simulink model "vacc_reorder"  (R2021a)
settings: Solver=VariableStepAuto  StartTime=0.0  StopTime=32*4*4+50  RelTol=1e-3
libraries: xbsIndex_r4 x285, casper_library_misc x2, casper_library_delays x2
(part 1 of 2)
settings Model: Creator=jackh  LastModifiedBy=vivado

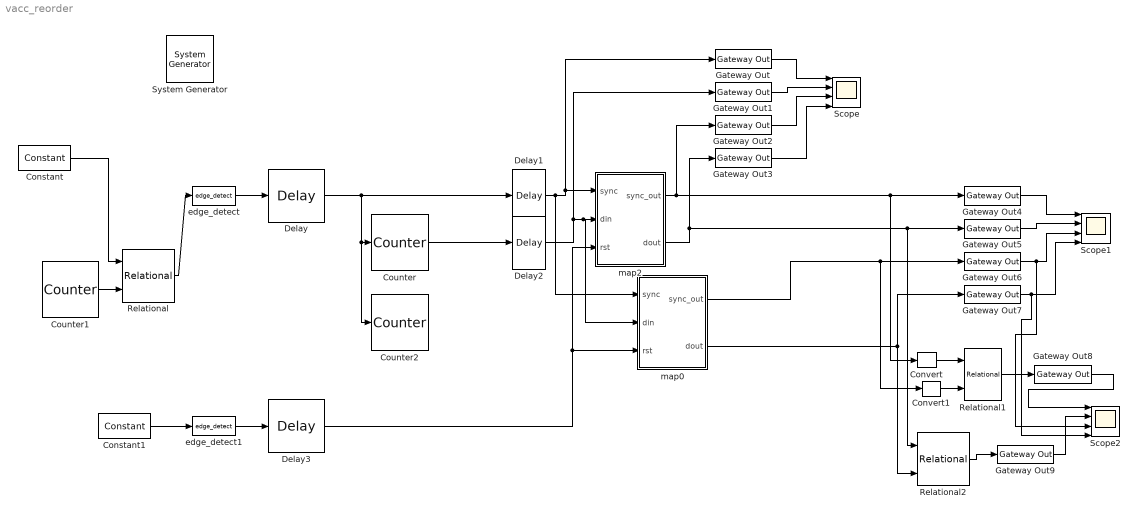
== system vacc_reorder ==
  " System Generator" : xbsIndex_r4/ System Generator  Tag=genX  xilinxfamily=zynquplusRFSOC  part=xczu47dr  speed=-2-e  package=ffvg1517  synthesis_tool=XST  clock_wrapper=Clock Enables  directory=/home/jackh/src/souk-firmware2/souk-firmware/firmware/src/souk_single_pipeline_krm/sysgen  proj_type=Vivado  Synth_file=Vivado Synthesis Defaults  Impl_file=Vivado Implementation Defaults  testbench=off  simulink_period=1  sysclk_period=3.2552  dcm_input_clock_period=10  incr_netlist=off  trim_vbits=Everywhere in SubSystem  dbl_ovrd=According to Block Masks  core_generation=According to Block Masks  run_coregen=off  deprecated_control=off  eval_field=0  block_type=sysgen
  Constant : xbsIndex_r4/Constant  const=0  gui_display_data_type=Fixed-point  arith_type=Unsigned  n_bits=7  bin_pt=0  preci_type=Single  exp_width=8  frac_width=24  explicit_period=on  period=1  equ=P=C  opselect=C  inp2=PCIN>>17  opr=+  inp1=P  carry=CIN  dbl_ovrd=off  block_type=constant
  Constant1 : xbsIndex_r4/Constant  const=1.0  gui_display_data_type=Boolean  arith_type=Boolean  n_bits=16  bin_pt=14  preci_type=Single  exp_width=8  frac_width=24  explicit_period=on  period=1  equ=P=C  opselect=C  inp2=PCIN>>17  opr=+  inp1=P  carry=CIN  dbl_ovrd=off  block_type=constant
  Convert : xbsIndex_r4/Convert  gui_display_data_type=Fixed-point  arith_type=Unsigned  n_bits=1  bin_pt=0  float_type=Single  exp_bits=8  fraction_bits=24  quantization=Truncate  overflow=Wrap  en=off  latency=0  pipeline=off  dbl_ovrd=off  block_type=convert
  Convert1 : xbsIndex_r4/Convert  gui_display_data_type=Fixed-point  arith_type=Unsigned  n_bits=1  bin_pt=0  float_type=Single  exp_bits=8  fraction_bits=24  quantization=Truncate  overflow=Wrap  en=off  latency=0  pipeline=off  dbl_ovrd=off  block_type=convert
  Counter : xbsIndex_r4/Counter  cnt_type=Count Limited  cnt_to=2^5 - 1  operation=Up  start_count=0  cnt_by_val=1  arith_type=Unsigned  n_bits=18*2*4  bin_pt=0  load_pin=off  rst=on  en=off  explicit_period=on  period=1  use_behavioral_HDL=off  implementation=Fabric  dbl_ovrd=off  block_type=counter
  Counter1 : xbsIndex_r4/Counter  cnt_type=Free Running  cnt_to=2^5 - 1  operation=Up  start_count=0  cnt_by_val=1  arith_type=Unsigned  n_bits=7  bin_pt=0  load_pin=off  rst=off  en=off  explicit_period=on  period=1  use_behavioral_HDL=off  implementation=Fabric  dbl_ovrd=off  block_type=counter
  Counter2 : xbsIndex_r4/Counter  cnt_type=Count Limited  cnt_to=0  operation=Down  start_count=2^6 - 1  cnt_by_val=1  arith_type=Unsigned  n_bits=18*2*4  bin_pt=0  load_pin=off  rst=on  en=off  explicit_period=on  period=1  use_behavioral_HDL=off  implementation=Fabric  dbl_ovrd=off  block_type=counter
  Delay : xbsIndex_r4/Delay  rst=off  infoeditControl=Selection of Reset will increase slice count due to use of real FFs and instead of SRLs  en=off  latency=50  reg_retiming=off  dbl_ovrd=off  block_type=delay
  Delay1 : xbsIndex_r4/Delay  rst=off  infoeditControl=Selection of Reset will increase slice count due to use of real FFs and instead of SRLs  en=off  latency=1  reg_retiming=off  dbl_ovrd=off  block_type=delay
  Delay2 : xbsIndex_r4/Delay  rst=off  infoeditControl=Selection of Reset will increase slice count due to use of real FFs and instead of SRLs  en=off  latency=1  reg_retiming=off  dbl_ovrd=off  block_type=delay
  Delay3 : xbsIndex_r4/Delay  rst=off  infoeditControl=Selection of Reset will increase slice count due to use of real FFs and instead of SRLs  en=off  latency=1  reg_retiming=off  dbl_ovrd=off  block_type=delay
  Gateway Out{,1..9} (10 alike) : xbsIndex_r4/Gateway Out  inherit_from_input=off  hdl_port=off  rows=1  columns=1  UseAsDAC=off  DACChannel='1'  interface=None  automatic_assignment=on  address_offset=hex2dec('00')  intf_name=''  intf_description=''  timing_constraint=None  locs_specified=off  LOCs={}  io_standard={}  block_type=gatewayout
  Relational : xbsIndex_r4/Relational  mode=a=b  op_type=Bool  en=off  latency=1  dbl_ovrd=off  block_type=relational
  Relational1 : xbsIndex_r4/Relational  mode=a=b  op_type=Bool  en=off  latency=0  dbl_ovrd=off  block_type=relational
  Relational2 : xbsIndex_r4/Relational  mode=a=b  op_type=Bool  en=off  latency=0  dbl_ovrd=off  block_type=relational
  Scope : Scope  NumInputPorts=4
  Scope1 : Scope  NumInputPorts=4
  Scope2 : Scope  NumInputPorts=4
  edge_detect : casper_library_misc/edge_detect  edge=Rising  polarity=Active High  x_in=[0 0.08 0.08 0.16 0.16 0.24 0.24 0.32 0.32 0.4]  y_in="[-1 -1  1  1  1  1  1  1  1  1]"  x_out=[0.6 0.68 0.68 0.76 0.76 0.84 0.84 0.92 0.92 1]  y_out="[-1 -1  1  1 -1 -1 -1 -1 -1 -1]"
  edge_detect1 : casper_library_misc/edge_detect  edge=Rising  polarity=Active High  x_in=[0 0.08 0.08 0.16 0.16 0.24 0.24 0.32 0.32 0.4]  y_in="[-1 -1  1  1  1  1  1  1  1  1]"  x_out=[0.6 0.68 0.68 0.76 0.76 0.84 0.84 0.92 0.92 1]  y_out="[-1 -1  1  1 -1 -1 -1 -1 -1 -1]"
  map0 : Subsystem  mask{vec_len_bits=5, ram_latency=2, sample_width=18, n_samples=4, add_latency=2}
      mask prompts: vec_len_bits "Vector length (2^?)"; ram_latency "Ram Latency"; sample_width "data width per sample"; n_samples "Number of samples per word"; add_latency "Adder latency"
  map2 : Subsystem  mask{vec_len_bits=5, ram_latency=2, sample_width=18, n_samples=4, add_latency=2}
      mask prompts: vec_len_bits "Vector length (2^?)"; ram_latency "Ram Latency"; sample_width "data width per sample"; n_samples "Number of samples per word"; add_latency "Adder latency"
  wires:
  edge_detect/1 -> Delay/1
  Delay/1 -> Counter2/1, Counter/1, Delay1/1
  Gateway Out1/1 -> Scope/2
  Gateway Out/1 -> Scope/1
  Gateway Out2/1 -> Scope/3
  Gateway Out3/1 -> Scope/4
  Counter1/1 -> Relational/2
  Relational/1 -> edge_detect/1
  Constant/1 -> Relational/1
  Delay1/1 -> map0/1(sync), map2/1(sync), Gateway Out/1
  Delay2/1 -> map0/2(din), map2/2(din), Gateway Out1/1
  Counter/1 -> Delay2/1
  Delay3/1 -> map0/3(rst), map2/3(rst)
  edge_detect1/1 -> Delay3/1
  Constant1/1 -> edge_detect1/1
  Gateway Out7/1 -> Scope2/4, Scope1/4
  Gateway Out6/1 -> Scope2/3, Scope1/3
  Gateway Out4/1 -> Scope1/1
  Gateway Out5/1 -> Scope1/2
  map2/1(sync_out) -> Gateway Out4/1, Convert/1, Gateway Out2/1
  map2/2(dout) -> Relational2/1, Gateway Out5/1, Gateway Out3/1
  Relational1/1 -> Gateway Out8/1
  Gateway Out8/1 -> Scope2/1
  Relational2/1 -> Gateway Out9/1
  Gateway Out9/1 -> Scope2/2
  Convert/1 -> Relational1/1
  Convert1/1 -> Relational1/2
  map0/2(dout) -> Gateway Out7/1, Relational2/2
  map0/1(sync_out) -> Convert1/1, Gateway Out6/1

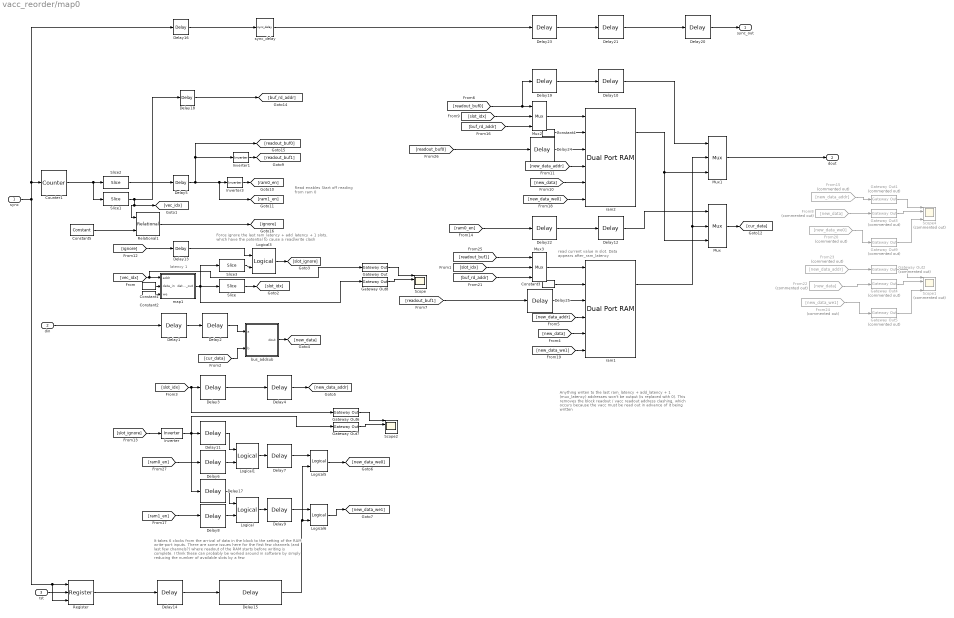
== system vacc_reorder/map0 ==
  note: Force ignore the last ram_latency + add_latency + 1 slots,
      | which have the potential to cause a read/write clash
  note: Anything writen to the last
      | ram_latency + add_latency + 1 (mux_latency)
      | addresses won't be output (is replaced with 0).
      | This removes the block readout / vacc readout address clashing,
      | which occurs because the vacc must be read out in advance of
      | it being written
  note: It takes 6 clocks from the arrival of data in the block
      | to the setting of the RAM write-port inputs. There are some issues
      | here for the first few channels (and last few channels?) where readout
      | of the RAM starts before writing is complete. I think these can probably
      | be worked around in software by simply reducing the number of available
      | slots by a few
  note: Read enables
      | Start off reading from ram 0
  note: read current value in slot.
      | Data appears after_ram_latency
  note: latency 1
  sync : Inport
  din : Inport  Port=2
  rst : Inport  Port=3
  Constant1 : xbsIndex_r4/Constant  const=0  gui_display_data_type=Fixed-point  arith_type=Unsigned  n_bits=32  bin_pt=0  preci_type=Single  exp_width=8  frac_width=24  explicit_period=on  period=1  equ=P=C  opselect=C  inp2=PCIN>>17  opr=+  inp1=P  carry=CIN  dbl_ovrd=off  block_type=constant
  Constant2 : xbsIndex_r4/Constant  const=0  gui_display_data_type=Boolean  arith_type=Boolean  n_bits=32  bin_pt=0  preci_type=Single  exp_width=8  frac_width=24  explicit_period=on  period=1  equ=P=C  opselect=C  inp2=PCIN>>17  opr=+  inp1=P  carry=CIN  dbl_ovrd=off  block_type=constant
  Constant3 : xbsIndex_r4/Constant  const=0  gui_display_data_type=Fixed-point  arith_type=Unsigned  n_bits=2*sample_width * n_samples  bin_pt=0  preci_type=Single  exp_width=8  frac_width=24  explicit_period=on  period=1  equ=P=C  opselect=C  inp2=PCIN>>17  opr=+  inp1=P  carry=CIN  dbl_ovrd=off  block_type=constant
  Constant4 : xbsIndex_r4/Constant  const=0  gui_display_data_type=Fixed-point  arith_type=Unsigned  n_bits=2*sample_width * n_samples  bin_pt=0  preci_type=Single  exp_width=8  frac_width=24  explicit_period=on  period=1  equ=P=C  opselect=C  inp2=PCIN>>17  opr=+  inp1=P  carry=CIN  dbl_ovrd=off  block_type=constant
  Constant5 : xbsIndex_r4/Constant  const="(2^vec_len_bits - 1) - (ram_latency + add_latency +  1 + 1 + 1+1)"  gui_display_data_type=Fixed-point  arith_type=Unsigned  n_bits=vec_len_bits  bin_pt=0  preci_type=Single  exp_width=8  frac_width=24  explicit_period=on  period=1  equ=P=C  opselect=C  inp2=PCIN>>17  opr=+  inp1=P  carry=CIN  dbl_ovrd=off  block_type=constant
  Counter1 : xbsIndex_r4/Counter  cnt_type=Free Running  cnt_to=Inf  operation=Up  start_count=0  cnt_by_val=1  arith_type=Unsigned  n_bits=vec_len_bits + 1  bin_pt=0  load_pin=off  rst=on  en=off  explicit_period=on  period=1  use_behavioral_HDL=off  implementation=Fabric  dbl_ovrd=off  block_type=counter
  Delay{1,5,13..14,16,18..20,22..25} (12 alike) : xbsIndex_r4/Delay  rst=off  infoeditControl=Selection of Reset will increase slice count due to use of real FFs and instead of SRLs  en=off  latency=1  reg_retiming=on  dbl_ovrd=off  block_type=delay
  Delay10 : xbsIndex_r4/Delay  rst=off  infoeditControl=Selection of Reset will increase slice count due to use of real FFs and instead of SRLs  en=off  latency=ram_latency  reg_retiming=on  dbl_ovrd=off  block_type=delay
  Delay11 : xbsIndex_r4/Delay  rst=off  infoeditControl=Selection of Reset will increase slice count due to use of real FFs and instead of SRLs  en=off  latency=1+1  reg_retiming=off  dbl_ovrd=off  block_type=delay
  Delay12 : xbsIndex_r4/Delay  rst=off  infoeditControl=Selection of Reset will increase slice count due to use of real FFs and instead of SRLs  en=off  latency=ram_latency  reg_retiming=on  dbl_ovrd=off  block_type=delay
  Delay15 : xbsIndex_r4/Delay  rst=off  infoeditControl=Selection of Reset will increase slice count due to use of real FFs and instead of SRLs  en=off  latency=ram_latency + add_latency +1+1  reg_retiming=on  dbl_ovrd=off  block_type=delay
  Delay17 : xbsIndex_r4/Delay  rst=off  infoeditControl=Selection of Reset will increase slice count due to use of real FFs and instead of SRLs  en=off  latency=1+1  reg_retiming=off  dbl_ovrd=off  block_type=delay
  Delay2 : xbsIndex_r4/Delay  rst=off  infoeditControl=Selection of Reset will increase slice count due to use of real FFs and instead of SRLs  en=off  latency=ram_latency+1+1  reg_retiming=on  dbl_ovrd=off  block_type=delay
  Delay21 : xbsIndex_r4/Delay  rst=off  infoeditControl=Selection of Reset will increase slice count due to use of real FFs and instead of SRLs  en=off  latency=ram_latency  reg_retiming=on  dbl_ovrd=off  block_type=delay
  Delay3 : xbsIndex_r4/Delay  rst=off  infoeditControl=Selection of Reset will increase slice count due to use of real FFs and instead of SRLs  en=off  latency=ram_latency+1+1  reg_retiming=on  dbl_ovrd=off  block_type=delay
  Delay4 : xbsIndex_r4/Delay  rst=off  infoeditControl=Selection of Reset will increase slice count due to use of real FFs and instead of SRLs  en=off  latency=add_latency  reg_retiming=on  dbl_ovrd=off  block_type=delay
  Delay6 : xbsIndex_r4/Delay  rst=off  infoeditControl=Selection of Reset will increase slice count due to use of real FFs and instead of SRLs  en=off  latency=1+1  reg_retiming=on  dbl_ovrd=off  block_type=delay
  Delay7 : xbsIndex_r4/Delay  rst=off  infoeditControl=Selection of Reset will increase slice count due to use of real FFs and instead of SRLs  en=off  latency=add_latency  reg_retiming=on  dbl_ovrd=off  block_type=delay
  Delay8 : xbsIndex_r4/Delay  rst=off  infoeditControl=Selection of Reset will increase slice count due to use of real FFs and instead of SRLs  en=off  latency=1+1  reg_retiming=on  dbl_ovrd=off  block_type=delay
  Delay9 : xbsIndex_r4/Delay  rst=off  infoeditControl=Selection of Reset will increase slice count due to use of real FFs and instead of SRLs  en=off  latency=add_latency  reg_retiming=on  dbl_ovrd=off  block_type=delay
  From15 : From  Commented=on  GotoTag=new_data_addr
  From20 : From  Commented=on  GotoTag=new_data_we0
  From22 : From  Commented=on  GotoTag=new_data
  From23 : From  Commented=on  GotoTag=new_data_addr
  From24 : From  Commented=on  GotoTag=new_data_we1
  From8 : From  Commented=on  GotoTag=new_data
  Gateway Out{,6..8} (4 alike) : xbsIndex_r4/Gateway Out  inherit_from_input=off  hdl_port=off  rows=1  columns=1  UseAsDAC=off  DACChannel='1'  interface=None  automatic_assignment=on  address_offset=hex2dec('00')  intf_name=''  intf_description=''  timing_constraint=None  locs_specified=off  LOCs={}  io_standard={}  block_type=gatewayout
  Gateway Out{1..5,9} (6 alike) : xbsIndex_r4/Gateway Out  Commented=on  inherit_from_input=off  hdl_port=off  rows=1  columns=1  UseAsDAC=off  DACChannel='1'  interface=None  automatic_assignment=on  address_offset=hex2dec('00')  intf_name=''  intf_description=''  timing_constraint=None  locs_specified=off  LOCs={}  io_standard={}  block_type=gatewayout
  Inverter : xbsIndex_r4/Inverter  en=off  latency=0  dbl_ovrd=off  block_type=inv
  Inverter1 : xbsIndex_r4/Inverter  en=off  latency=0  dbl_ovrd=off  block_type=inv
  Inverter3 : xbsIndex_r4/Inverter  en=off  latency=0  dbl_ovrd=off  block_type=inv
  Logical : xbsIndex_r4/Logical  logical_function=AND  inputs=2  en=off  latency=ram_latency  precision=Full  arith_type=Unsigned  n_bits=16  bin_pt=0  align_bp=on  dbl_ovrd=off  block_type=logical
  Logical1 : xbsIndex_r4/Logical  logical_function=AND  inputs=2  en=off  latency=ram_latency  precision=Full  arith_type=Unsigned  n_bits=16  bin_pt=0  align_bp=on  dbl_ovrd=off  block_type=logical
  Logical3 : xbsIndex_r4/Logical  logical_function=OR  inputs=2  en=off  latency=0  precision=Full  arith_type=Unsigned  n_bits=16  bin_pt=0  align_bp=on  dbl_ovrd=off  block_type=logical
  Logical5 : xbsIndex_r4/Logical  logical_function=AND  inputs=2  en=off  latency=0  precision=Full  arith_type=Unsigned  n_bits=16  bin_pt=0  align_bp=on  dbl_ovrd=off  block_type=logical
  Logical6 : xbsIndex_r4/Logical  logical_function=AND  inputs=2  en=off  latency=0  precision=Full  arith_type=Unsigned  n_bits=16  bin_pt=0  align_bp=on  dbl_ovrd=off  block_type=logical
  Mux{,1..3} (4 alike) : xbsIndex_r4/Mux  inputs=2  en=off  latency=1  precision=Full  arith_type=Unsigned  n_bits=16  bin_pt=14  quantization=Truncate  overflow=Wrap  dbl_ovrd=off  block_type=mux
  Register : xbsIndex_r4/Register  init=0  rst=on  en=on  dbl_ovrd=off  block_type=register
  Relational1 : xbsIndex_r4/Relational  mode=a>b  op_type=Bool  en=off  latency=0  dbl_ovrd=off  block_type=relational
  Scope : Scope  NumInputPorts=4
  Scope1 : Scope  Commented=on  NumInputPorts=4
  Scope2 : Scope  NumInputPorts=4
  Scope4 : Scope  Commented=on  NumInputPorts=4
  Slice : xbsIndex_r4/Slice  nbits=vec_len_bits  boolean_output=off  mode=Lower Bit Location + Width  bit1=0  base1=MSB of Input  bit0=0  base0=LSB of Input  dbl_ovrd=off  block_type=slice
  Slice1 : xbsIndex_r4/Slice  nbits=vec_len_bits  boolean_output=off  mode=Lower Bit Location + Width  bit1=0  base1=MSB of Input  bit0=0  base0=LSB of Input  dbl_ovrd=off  block_type=slice
  Slice2 : xbsIndex_r4/Slice  nbits=1  boolean_output=on  mode=Lower Bit Location + Width  bit1=0  base1=MSB of Input  bit0=vec_len_bits  base0=LSB of Input  dbl_ovrd=off  block_type=slice
  Slice3 : xbsIndex_r4/Slice  nbits=1  boolean_output=on  mode=Upper Bit Location + Width  bit1=0  base1=MSB of Input  bit0=0  base0=LSB of Input  dbl_ovrd=off  block_type=slice
  bus_addsub : Subsystem  AncestorBlock=casper_library_bus/bus_addsub  mask(bus_addsub){opmode=0, n_bits_a=sample_width*ones(n_samples,1), bin_pt_a=zeros(n_samples,1), type_a=1, n_bits_b=sample_width*ones(n_samples,1), bin_pt_b=zeros(n_samples,1), type_b=1, cmplx=on, misc=off, async=off, floating_point=off, float_type=single, exp_width=6, frac_width=19, n_bits_out=sample_width*ones(n_samples,1), bin_pt_out=zeros(n_samples,1), type_out=1, quantization=0, overflow=1, add_implementation=behavioral HDL, csp_latency=add_latency, pipeline_en=off, pipeline_latency=0}
      mask prompts: opmode "mode (Addition=0, Subtraction=1)"; n_bits_a "a input bit widths"; bin_pt_a "a input binary points"; type_a "a input type (Unsigned=0, Signed=1)"; n_bits_b "b input bit widths"; bin_pt_b "b input binary points"; type_b "b input type (Unsigned=0, Signed=1)"; cmplx "complex"; misc "misc support"; async "asynchronous operation"; floating_point "floating point"; exp_width "exponent width"; frac_width "fraction width"; n_bits_out "output bit widths"; bin_pt_out "output binary points"; type_out "output type (Unsigned=0, Signed=1)"; quantization "quantization strategy (Truncate=0, Round  (unbiased: +/- Inf)=1)"; overflow "overflow strategy (Wrap=0, Saturate=1, Flag as error=2)"; add_implementation "adder implementation"; csp_latency "latency"; pipeline_en "pipeline enable"; pipeline_latency "pipeline latency"
      mask help: Add/subtract components of two busses
      mask init:
      | bus_addsub_init(gcb, ...
      |     'opmode', opmode, ...
      |     'n_bits_a', n_bits_a, ...
      |     'bin_pt_a', bin_pt_a, ...
      |     'type_a', type_a, ...
      |     'n_bits_b', n_bits_b, ...
      |     'bin_pt_b', bin_pt_b, ...
      |     'type_b', type_b, ...
      |     'n_bits_out', n_bits_out, ...
      |     'bin_pt_out', bin_pt_out, ...
      |     'floating_point', floating_point, ...
      |     'float_type', float_type, ...
      |     'exp_width', exp_width, ...
      |     'frac_width', frac_width, ...
      |     'type_out', type_out, ...
      |     'overflow', overflow, ...        
      |     'quantization', quantization, ...
      |     'add_implementation', add_implementation, ...
      |     'csp_latency', csp_latency, ...
      |     'pipeline_en', pipeline_en, ...
      |     'pipeline_latency', pipeline_latency,...
      |     'cmplx', cmplx, ...
      |     'misc', misc, ...
      |     'async', async);
      mask Callback floating_point:
      | onoff = get_param(gcb, 'floating_point');
      | if strcmp(onoff,'on')
      |     enable_fixpt = 'off';
      |     set_param_state(gcb, 'float_type', 'on')
      | 
      |     f_type = get_param(gcb, 'float_type');
      |     if strcmp(f_type,'custom')
      |         set_param_state(gcb, 'exp_width', 'on')
      |         set_param_state(gcb, 'frac_width', 'on')
      |     else
      |         set_param_state(gcb, 'exp_width', 'off')
      |         set_param_state(gcb, 'frac_width', 'off')
      |     end
      | 
      | 
      | else
      |     enable_fixpt = 'on';
      |     set_param_state(gcb, 'float_type', 'off')
      |     set_param_state(gcb, 'exp_width', 'off')
      |     set_param_state(gcb, 'frac_width', 'off')
      | end
      | 
      | set_param_state(gcb, 'n_bits_a', enable_fixpt)
      | set_param_state(gcb, 'bin_pt_a', enable_fixpt)
      | set_param_state(gcb, 'type_a', enable_fixpt)
      | set_param_state(gcb, 'n_bits_b', enable_fixpt)
      | set_param_state(gcb, 'bin_pt_b', enable_fixpt)
      | set_param_state(gcb, 'type_b', enable_fixpt)
      | 
      | set_param_state(gcb, 'n_bits_out', enable_fixpt)
      | set_param_state(gcb, 'bin_pt_out', enable_fixpt)
      | set_param_state(gcb, 'type_out', enable_fixpt)
      | set_param_state(gcb, 'quantization', enable_fixpt)
      | set_param_state(gcb, 'overflow', enable_fixpt)
      mask TypeOptions float_type: single | custom
      mask Callback float_type:
      | f_type = get_param(gcb, 'float_type');
      | if strcmp(f_type,'custom')
      |     set_param_state(gcb, 'exp_width', 'on')
      |     set_param_state(gcb, 'frac_width', 'on')
      | else
      |     set_param_state(gcb, 'exp_width', 'off')
      |     set_param_state(gcb, 'frac_width', 'off')
      | end
      mask TypeOptions add_implementation: behavioral HDL | fabric core | DSP48 core
  map1 : Subsystem  Tag=xps:bram  AncestorBlock=xps_library/Memory/shared_bram  mask{arith_type=Unsigned, addr_width=vec_len_bits, data_width=16, reg_prim_output=off, reg_core_output=off, optimization=Minimum_Area, data_bin_pt=0, init_vals=[2^vec_len_bits-1:-1:0], sample_rate=1, desc_str="", type_desc='uint32'}
      mask prompts: arith_type "Output Data Type"; addr_width "Address width"; data_width "Data Width"; reg_prim_output "Register Primitive Output"; reg_core_output "Register Core Output"; data_bin_pt "Data Binary Point"; init_vals "Initial values (simulation only)"; sample_rate "Sample rate"; desc_str "Description"; type_desc "Data Type Description"
      mask init:
      | shared_bram_mask;
      mask TypeOptions arith_type: Unsigned | Signed  (2's comp)
      mask TypeOptions data_width: 8 | 16 | 32 | 64 | 128 | 256 | 512 | 1024
      mask TypeOptions optimization: Minimum_Area | Low_Power
  ram1 : xbsIndex_r4/Dual Port RAM  depth=2^vec_len_bits  initVector=zeros(1,2^vec_len_bits)  distributed_mem=Block RAM  init_a=0  init_b=0  rst_a=off  rst_b=off  en_a=off  en_b=off  latency=ram_latency  write_mode_A=Read Before Write  write_mode_B=Read Before Write  optimize=Area  dbl_ovrd=off  simulation_type=fast_sim  block_type=dpram
  ram2 : xbsIndex_r4/Dual Port RAM  depth=2^vec_len_bits  initVector=zeros(1,2^vec_len_bits)  distributed_mem=Block RAM  init_a=0  init_b=0  rst_a=off  rst_b=off  en_a=off  en_b=off  latency=ram_latency  write_mode_A=Read Before Write  write_mode_B=Read Before Write  optimize=Area  dbl_ovrd=off  simulation_type=fast_sim  block_type=dpram
  sync_delay : casper_library_delays/sync_delay  DelayLen=2^vec_len_bits
      settings: SourceProductName=CASPER DSP Blockset
  sync_out : Outport
  dout : Outport  Port=2
  wires:
  Delay25/1 -> ram1/3
  Delay24/1 -> ram2/3
  Delay23/1 -> Delay21/1
  Delay22/1 -> Delay12/1
  Delay19/1 -> Delay10/1
  Gateway Out8/1 -> Scope/2
  ? -> Scope/4
  Gateway Out/1 -> Scope/1
  ? -> Scope/3
  Delay18/1 -> [buf_rd_addr]
  From20/1 -> Gateway Out9/1
  From8/1 -> Gateway Out3/1
  From15/1 -> Gateway Out1/1
  Gateway Out9/1 -> Scope4/4
  Gateway Out3/1 -> Scope4/2
  ? -> Scope4/3
  Gateway Out1/1 -> Scope4/1
  Delay16/1 -> sync_delay/1
  Inverter1/1 -> [readout_buf1]
  Relational1/1 -> [ignore]
  Constant5/1 -> Relational1/2
  Inverter3/1 -> [ram0_en]
  map1/1(data_out) -> Slice3/1, Slice/1, Gateway Out8/1
  Counter1/1 -> Slice2/1, Slice1/1
  Slice1/1 -> [vec_idx], Relational1/1, Delay18/1
  [vec_idx] -> map1/1(addr), Gateway Out/1
  Constant1/1 -> map1/2(data_in)
  Constant2/1 -> map1/3(we)
  din/1 -> Delay1/1
  Slice/1 -> [slot_idx]
  Delay1/1 -> Delay2/1
  [cur_data] -> bus_addsub/2(b)
  Delay2/1 -> bus_addsub/1(a)
  Delay3/1 -> Delay4/1
  bus_addsub/1(dout) -> [new_data]
  Delay4/1 -> [new_data_addr]
  Slice2/1 -> Delay5/1
  ram2/1 -> Mux/3, Mux1/3
  [readout_buf0] -> Delay24/1
  Mux/1 -> [cur_data]
  Mux2/1 -> ram2/1
  [buf_rd_addr] -> Mux2/3
  [slot_idx] -> Mux2/2
  [slot_idx] -> Mux3/2
  [buf_rd_addr] -> Mux3/3
  Mux3/1 -> ram1/1
  Constant3/1 -> ram1/2
  Constant4/1 -> ram2/2
  ram1/1 -> Mux1/2, Mux/2
  [ram0_en] -> Delay6/1
  [ram1_en] -> Delay8/1
  [new_data] -> ram1/5
  [new_data_addr] -> ram1/4
  [new_data_we1] -> ram1/6
  [ram0_en] -> Delay22/1
  Delay12/1 -> Mux/1
  [readout_buf1] -> Delay25/1
  Mux1/1 -> dout/1
  Delay20/1 -> sync_out/1
  Delay21/1 -> Delay20/1
  sync_delay/1 -> Delay23/1
  sync/1 -> Register/3, Register/1, Counter1/1, Delay16/1
  [new_data_addr] -> ram2/4
  [new_data_we0] -> ram2/6
  [new_data] -> ram2/5
  [slot_ignore] -> Inverter/1
  Inverter/1 -> Gateway Out7/1, Delay17/1, Delay11/1
  Delay8/1 -> Logical/2
  Logical/1 -> Delay9/1
  Delay17/1 -> Logical/1
  Delay6/1 -> Logical1/2
  Delay11/1 -> Logical1/1
  Logical1/1 -> Delay7/1
  Logical3/1 -> [slot_ignore]
  [ignore] -> Delay13/1
  Slice3/1 -> Logical3/2
  Gateway Out2/1 -> Scope1/1
  ? -> Scope1/3
  Gateway Out4/1 -> Scope1/2
  Gateway Out5/1 -> Scope1/4
  From23/1 -> Gateway Out2/1
  From22/1 -> Gateway Out4/1
  From24/1 -> Gateway Out5/1
  Delay13/1 -> Logical3/1
  [slot_idx] -> Gateway Out6/1, Delay3/1
  Gateway Out7/1 -> Scope2/2
  Gateway Out6/1 -> Scope2/1
  rst/1 -> Register/2
  Register/1 -> Delay14/1
  Delay14/1 -> Delay15/1
  Delay7/1 -> Logical5/1
  Logical5/1 -> [new_data_we0]
  Delay9/1 -> Logical6/1
  Logical6/1 -> [new_data_we1]
  Delay15/1 -> Logical5/2, Logical6/2
  Delay5/1 -> Inverter3/1, [ram1_en], [readout_buf0], Inverter1/1
  [readout_buf0] -> Delay19/1, Mux2/1
  Delay10/1 -> Mux1/1
  [readout_buf1] -> Mux3/1

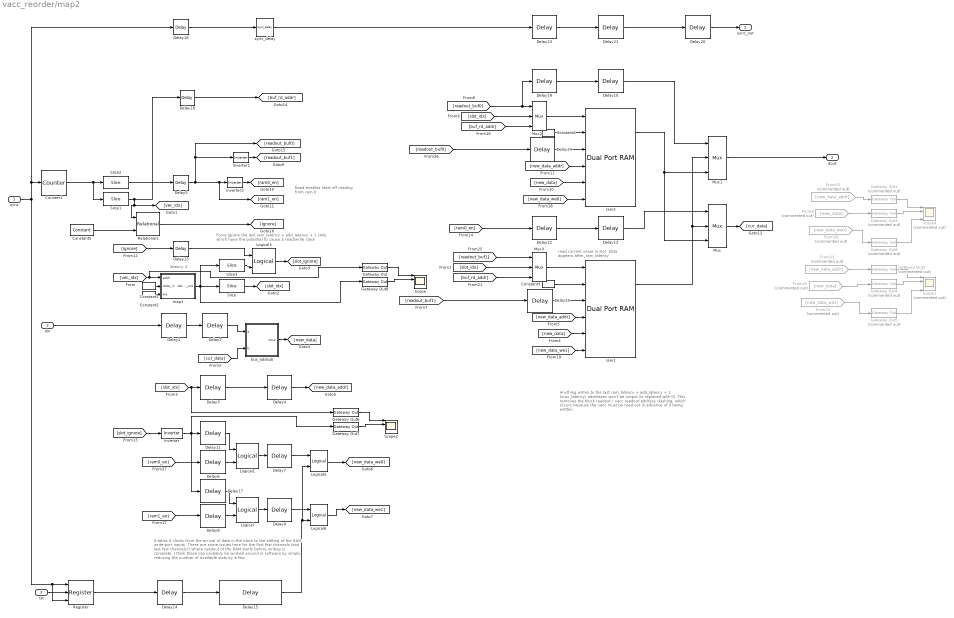
== system vacc_reorder/map2 ==
  note: latency 2
  note: read current value in slot.
      | Data appears after_ram_latency
  note: Read enables
      | Start off reading from ram 0
  note: It takes 6 clocks from the arrival of data in the block
      | to the setting of the RAM write-port inputs. There are some issues
      | here for the first few channels (and last few channels?) where readout
      | of the RAM starts before writing is complete. I think these can probably
      | be worked around in software by simply reducing the number of available
      | slots by a few
  note: Anything writen to the last
      | ram_latency + add_latency + 1 (mux_latency)
      | addresses won't be output (is replaced with 0).
      | This removes the block readout / vacc readout address clashing,
      | which occurs because the vacc must be read out in advance of
      | it being written
  note: Force ignore the last ram_latency + add_latency + 1 slots,
      | which have the potential to cause a read/write clash
  sync : Inport
  din : Inport  Port=2
  rst : Inport  Port=3
  Constant1 : xbsIndex_r4/Constant  const=0  gui_display_data_type=Fixed-point  arith_type=Unsigned  n_bits=32  bin_pt=0  preci_type=Single  exp_width=8  frac_width=24  explicit_period=on  period=1  equ=P=C  opselect=C  inp2=PCIN>>17  opr=+  inp1=P  carry=CIN  dbl_ovrd=off  block_type=constant
  Constant2 : xbsIndex_r4/Constant  const=0  gui_display_data_type=Boolean  arith_type=Boolean  n_bits=32  bin_pt=0  preci_type=Single  exp_width=8  frac_width=24  explicit_period=on  period=1  equ=P=C  opselect=C  inp2=PCIN>>17  opr=+  inp1=P  carry=CIN  dbl_ovrd=off  block_type=constant
  Constant3 : xbsIndex_r4/Constant  const=0  gui_display_data_type=Fixed-point  arith_type=Unsigned  n_bits=2*sample_width * n_samples  bin_pt=0  preci_type=Single  exp_width=8  frac_width=24  explicit_period=on  period=1  equ=P=C  opselect=C  inp2=PCIN>>17  opr=+  inp1=P  carry=CIN  dbl_ovrd=off  block_type=constant
  Constant4 : xbsIndex_r4/Constant  const=0  gui_display_data_type=Fixed-point  arith_type=Unsigned  n_bits=2*sample_width * n_samples  bin_pt=0  preci_type=Single  exp_width=8  frac_width=24  explicit_period=on  period=1  equ=P=C  opselect=C  inp2=PCIN>>17  opr=+  inp1=P  carry=CIN  dbl_ovrd=off  block_type=constant
  Constant5 : xbsIndex_r4/Constant  const="(2^vec_len_bits - 1) - (ram_latency + add_latency +  1 + 1 + 1+1)"  gui_display_data_type=Fixed-point  arith_type=Unsigned  n_bits=vec_len_bits  bin_pt=0  preci_type=Single  exp_width=8  frac_width=24  explicit_period=on  period=1  equ=P=C  opselect=C  inp2=PCIN>>17  opr=+  inp1=P  carry=CIN  dbl_ovrd=off  block_type=constant
  Counter1 : xbsIndex_r4/Counter  cnt_type=Free Running  cnt_to=Inf  operation=Up  start_count=0  cnt_by_val=1  arith_type=Unsigned  n_bits=vec_len_bits + 1  bin_pt=0  load_pin=off  rst=on  en=off  explicit_period=on  period=1  use_behavioral_HDL=off  implementation=Fabric  dbl_ovrd=off  block_type=counter
  Delay{1,5..6,8,13..14,16,18..20,22..25} (14 alike) : xbsIndex_r4/Delay  rst=off  infoeditControl=Selection of Reset will increase slice count due to use of real FFs and instead of SRLs  en=off  latency=1  reg_retiming=on  dbl_ovrd=off  block_type=delay
  Delay10 : xbsIndex_r4/Delay  rst=off  infoeditControl=Selection of Reset will increase slice count due to use of real FFs and instead of SRLs  en=off  latency=ram_latency  reg_retiming=on  dbl_ovrd=off  block_type=delay
  Delay11 : xbsIndex_r4/Delay  rst=off  infoeditControl=Selection of Reset will increase slice count due to use of real FFs and instead of SRLs  en=off  latency=1  reg_retiming=off  dbl_ovrd=off  block_type=delay
  Delay12 : xbsIndex_r4/Delay  rst=off  infoeditControl=Selection of Reset will increase slice count due to use of real FFs and instead of SRLs  en=off  latency=ram_latency  reg_retiming=on  dbl_ovrd=off  block_type=delay
  Delay15 : xbsIndex_r4/Delay  rst=off  infoeditControl=Selection of Reset will increase slice count due to use of real FFs and instead of SRLs  en=off  latency=ram_latency + add_latency +1  reg_retiming=on  dbl_ovrd=off  block_type=delay
  Delay17 : xbsIndex_r4/Delay  rst=off  infoeditControl=Selection of Reset will increase slice count due to use of real FFs and instead of SRLs  en=off  latency=1  reg_retiming=off  dbl_ovrd=off  block_type=delay
  Delay2 : xbsIndex_r4/Delay  rst=off  infoeditControl=Selection of Reset will increase slice count due to use of real FFs and instead of SRLs  en=off  latency=ram_latency+1  reg_retiming=on  dbl_ovrd=off  block_type=delay
  Delay21 : xbsIndex_r4/Delay  rst=off  infoeditControl=Selection of Reset will increase slice count due to use of real FFs and instead of SRLs  en=off  latency=ram_latency  reg_retiming=on  dbl_ovrd=off  block_type=delay
  Delay3 : xbsIndex_r4/Delay  rst=off  infoeditControl=Selection of Reset will increase slice count due to use of real FFs and instead of SRLs  en=off  latency=ram_latency+1  reg_retiming=on  dbl_ovrd=off  block_type=delay
  Delay4 : xbsIndex_r4/Delay  rst=off  infoeditControl=Selection of Reset will increase slice count due to use of real FFs and instead of SRLs  en=off  latency=add_latency  reg_retiming=on  dbl_ovrd=off  block_type=delay
  Delay7 : xbsIndex_r4/Delay  rst=off  infoeditControl=Selection of Reset will increase slice count due to use of real FFs and instead of SRLs  en=off  latency=add_latency  reg_retiming=on  dbl_ovrd=off  block_type=delay
  Delay9 : xbsIndex_r4/Delay  rst=off  infoeditControl=Selection of Reset will increase slice count due to use of real FFs and instead of SRLs  en=off  latency=add_latency  reg_retiming=on  dbl_ovrd=off  block_type=delay
  From15 : From  Commented=on  GotoTag=new_data_addr
  From20 : From  Commented=on  GotoTag=new_data_we0
  From22 : From  Commented=on  GotoTag=new_data
  From23 : From  Commented=on  GotoTag=new_data_addr
  From24 : From  Commented=on  GotoTag=new_data_we1
  From8 : From  Commented=on  GotoTag=new_data
  Gateway Out{,6..8} (4 alike) : xbsIndex_r4/Gateway Out  inherit_from_input=off  hdl_port=off  rows=1  columns=1  UseAsDAC=off  DACChannel='1'  interface=None  automatic_assignment=on  address_offset=hex2dec('00')  intf_name=''  intf_description=''  timing_constraint=None  locs_specified=off  LOCs={}  io_standard={}  block_type=gatewayout
  Gateway Out{1..5,9} (6 alike) : xbsIndex_r4/Gateway Out  Commented=on  inherit_from_input=off  hdl_port=off  rows=1  columns=1  UseAsDAC=off  DACChannel='1'  interface=None  automatic_assignment=on  address_offset=hex2dec('00')  intf_name=''  intf_description=''  timing_constraint=None  locs_specified=off  LOCs={}  io_standard={}  block_type=gatewayout
  Inverter : xbsIndex_r4/Inverter  en=off  latency=0  dbl_ovrd=off  block_type=inv
  Inverter1 : xbsIndex_r4/Inverter  en=off  latency=0  dbl_ovrd=off  block_type=inv
  Inverter3 : xbsIndex_r4/Inverter  en=off  latency=0  dbl_ovrd=off  block_type=inv
  Logical : xbsIndex_r4/Logical  logical_function=AND  inputs=2  en=off  latency=ram_latency  precision=Full  arith_type=Unsigned  n_bits=16  bin_pt=0  align_bp=on  dbl_ovrd=off  block_type=logical
  Logical1 : xbsIndex_r4/Logical  logical_function=AND  inputs=2  en=off  latency=ram_latency  precision=Full  arith_type=Unsigned  n_bits=16  bin_pt=0  align_bp=on  dbl_ovrd=off  block_type=logical
  Logical3 : xbsIndex_r4/Logical  logical_function=OR  inputs=2  en=off  latency=0  precision=Full  arith_type=Unsigned  n_bits=16  bin_pt=0  align_bp=on  dbl_ovrd=off  block_type=logical
  Logical5 : xbsIndex_r4/Logical  logical_function=AND  inputs=2  en=off  latency=0  precision=Full  arith_type=Unsigned  n_bits=16  bin_pt=0  align_bp=on  dbl_ovrd=off  block_type=logical
  Logical6 : xbsIndex_r4/Logical  logical_function=AND  inputs=2  en=off  latency=0  precision=Full  arith_type=Unsigned  n_bits=16  bin_pt=0  align_bp=on  dbl_ovrd=off  block_type=logical
  Mux{,1..3} (4 alike) : xbsIndex_r4/Mux  inputs=2  en=off  latency=1  precision=Full  arith_type=Unsigned  n_bits=16  bin_pt=14  quantization=Truncate  overflow=Wrap  dbl_ovrd=off  block_type=mux
  Register : xbsIndex_r4/Register  init=0  rst=on  en=on  dbl_ovrd=off  block_type=register
  Relational1 : xbsIndex_r4/Relational  mode=a>b  op_type=Bool  en=off  latency=0  dbl_ovrd=off  block_type=relational
  Scope : Scope  NumInputPorts=4
  Scope1 : Scope  Commented=on  NumInputPorts=4
  Scope2 : Scope  NumInputPorts=4
  Scope4 : Scope  Commented=on  NumInputPorts=4
  Slice : xbsIndex_r4/Slice  nbits=vec_len_bits  boolean_output=off  mode=Lower Bit Location + Width  bit1=0  base1=MSB of Input  bit0=0  base0=LSB of Input  dbl_ovrd=off  block_type=slice
  Slice1 : xbsIndex_r4/Slice  nbits=vec_len_bits  boolean_output=off  mode=Lower Bit Location + Width  bit1=0  base1=MSB of Input  bit0=0  base0=LSB of Input  dbl_ovrd=off  block_type=slice
  Slice2 : xbsIndex_r4/Slice  nbits=1  boolean_output=on  mode=Lower Bit Location + Width  bit1=0  base1=MSB of Input  bit0=vec_len_bits  base0=LSB of Input  dbl_ovrd=off  block_type=slice
  Slice3 : xbsIndex_r4/Slice  nbits=1  boolean_output=on  mode=Upper Bit Location + Width  bit1=0  base1=MSB of Input  bit0=0  base0=LSB of Input  dbl_ovrd=off  block_type=slice
  bus_addsub : Subsystem  AncestorBlock=casper_library_bus/bus_addsub  mask(bus_addsub){opmode=0, n_bits_a=sample_width*ones(n_samples,1), bin_pt_a=zeros(n_samples,1), type_a=1, n_bits_b=sample_width*ones(n_samples,1), bin_pt_b=zeros(n_samples,1), type_b=1, cmplx=on, misc=off, async=off, floating_point=off, float_type=single, exp_width=6, frac_width=19, n_bits_out=sample_width*ones(n_samples,1), bin_pt_out=zeros(n_samples,1), type_out=1, quantization=0, overflow=1, add_implementation=behavioral HDL, csp_latency=add_latency, pipeline_en=off, pipeline_latency=0}
      mask prompts: opmode "mode (Addition=0, Subtraction=1)"; n_bits_a "a input bit widths"; bin_pt_a "a input binary points"; type_a "a input type (Unsigned=0, Signed=1)"; n_bits_b "b input bit widths"; bin_pt_b "b input binary points"; type_b "b input type (Unsigned=0, Signed=1)"; cmplx "complex"; misc "misc support"; async "asynchronous operation"; floating_point "floating point"; exp_width "exponent width"; frac_width "fraction width"; n_bits_out "output bit widths"; bin_pt_out "output binary points"; type_out "output type (Unsigned=0, Signed=1)"; quantization "quantization strategy (Truncate=0, Round  (unbiased: +/- Inf)=1)"; overflow "overflow strategy (Wrap=0, Saturate=1, Flag as error=2)"; add_implementation "adder implementation"; csp_latency "latency"; pipeline_en "pipeline enable"; pipeline_latency "pipeline latency"
      mask help: Add/subtract components of two busses
      mask init: same as vacc_reorder/map0/bus_addsub
      mask Callback floating_point:
      | onoff = get_param(gcb, 'floating_point');
      | if strcmp(onoff,'on')
      |     enable_fixpt = 'off';
      |     set_param_state(gcb, 'float_type', 'on')
      | 
      |     f_type = get_param(gcb, 'float_type');
      |     if strcmp(f_type,'custom')
      |         set_param_state(gcb, 'exp_width', 'on')
      |         set_param_state(gcb, 'frac_width', 'on')
      |     else
      |         set_param_state(gcb, 'exp_width', 'off')
      |         set_param_state(gcb, 'frac_width', 'off')
      |     end
      | 
      | 
      | else
      |     enable_fixpt = 'on';
      |     set_param_state(gcb, 'float_type', 'off')
      |     set_param_state(gcb, 'exp_width', 'off')
      |     set_param_state(gcb, 'frac_width', 'off')
      | end
      | 
      | set_param_state(gcb, 'n_bits_a', enable_fixpt)
      | set_param_state(gcb, 'bin_pt_a', enable_fixpt)
      | set_param_state(gcb, 'type_a', enable_fixpt)
      | set_param_state(gcb, 'n_bits_b', enable_fixpt)
      | set_param_state(gcb, 'bin_pt_b', enable_fixpt)
      | set_param_state(gcb, 'type_b', enable_fixpt)
      | 
      | set_param_state(gcb, 'n_bits_out', enable_fixpt)
      | set_param_state(gcb, 'bin_pt_out', enable_fixpt)
      | set_param_state(gcb, 'type_out', enable_fixpt)
      | set_param_state(gcb, 'quantization', enable_fixpt)
      | set_param_state(gcb, 'overflow', enable_fixpt)
      mask TypeOptions float_type: single | custom
      mask Callback float_type:
      | f_type = get_param(gcb, 'float_type');
      | if strcmp(f_type,'custom')
      |     set_param_state(gcb, 'exp_width', 'on')
      |     set_param_state(gcb, 'frac_width', 'on')
      | else
      |     set_param_state(gcb, 'exp_width', 'off')
      |     set_param_state(gcb, 'frac_width', 'off')
      | end
      mask TypeOptions add_implementation: behavioral HDL | fabric core | DSP48 core
  map1 : Subsystem  Tag=xps:bram  AncestorBlock=xps_library/Memory/shared_bram  mask{arith_type=Unsigned, addr_width=vec_len_bits, data_width=16, reg_prim_output=off, reg_core_output=off, optimization=Minimum_Area, data_bin_pt=0, init_vals=[2^vec_len_bits-1:-1:0], sample_rate=1, desc_str="", type_desc='uint32'}
      mask prompts: arith_type "Output Data Type"; addr_width "Address width"; data_width "Data Width"; reg_prim_output "Register Primitive Output"; reg_core_output "Register Core Output"; data_bin_pt "Data Binary Point"; init_vals "Initial values (simulation only)"; sample_rate "Sample rate"; desc_str "Description"; type_desc "Data Type Description"
      mask init:
      | shared_bram_mask;
      mask TypeOptions arith_type: Unsigned | Signed  (2's comp)
      mask TypeOptions data_width: 8 | 16 | 32 | 64 | 128 | 256 | 512 | 1024
      mask TypeOptions optimization: Minimum_Area | Low_Power
  ram1 : xbsIndex_r4/Dual Port RAM  depth=2^vec_len_bits  initVector=zeros(1,2^vec_len_bits)  distributed_mem=Block RAM  init_a=0  init_b=0  rst_a=off  rst_b=off  en_a=off  en_b=off  latency=ram_latency  write_mode_A=Read Before Write  write_mode_B=Read Before Write  optimize=Area  dbl_ovrd=off  simulation_type=fast_sim  block_type=dpram
  ram2 : xbsIndex_r4/Dual Port RAM  depth=2^vec_len_bits  initVector=zeros(1,2^vec_len_bits)  distributed_mem=Block RAM  init_a=0  init_b=0  rst_a=off  rst_b=off  en_a=off  en_b=off  latency=ram_latency  write_mode_A=Read Before Write  write_mode_B=Read Before Write  optimize=Area  dbl_ovrd=off  simulation_type=fast_sim  block_type=dpram
  sync_delay : casper_library_delays/sync_delay  DelayLen=2^vec_len_bits
      settings: SourceProductName=CASPER DSP Blockset
  sync_out : Outport
  dout : Outport  Port=2
  wires:
  [readout_buf1] -> Mux3/1
  Delay10/1 -> Mux1/1
  [readout_buf0] -> Mux2/1, Delay19/1
  Delay5/1 -> Inverter1/1, [readout_buf0], [ram1_en], Inverter3/1
  Delay15/1 -> Logical6/2, Logical5/2
  Logical6/1 -> [new_data_we1]
  Delay9/1 -> Logical6/1
  Logical5/1 -> [new_data_we0]
  Delay7/1 -> Logical5/1
  Delay14/1 -> Delay15/1
  Register/1 -> Delay14/1
  rst/1 -> Register/2
  Gateway Out6/1 -> Scope2/1
  Gateway Out7/1 -> Scope2/2
  [slot_idx] -> Delay3/1, Gateway Out6/1
  Delay13/1 -> Logical3/1
  From24/1 -> Gateway Out5/1
  From22/1 -> Gateway Out4/1
  From23/1 -> Gateway Out2/1
  Gateway Out5/1 -> Scope1/4
  Gateway Out4/1 -> Scope1/2
  ? -> Scope1/3
  Gateway Out2/1 -> Scope1/1
  Slice3/1 -> Logical3/2
  [ignore] -> Delay13/1
  Logical3/1 -> [slot_ignore]
  Logical1/1 -> Delay7/1
  Delay11/1 -> Logical1/1
  Delay6/1 -> Logical1/2
  Delay17/1 -> Logical/1
  Logical/1 -> Delay9/1
  Delay8/1 -> Logical/2
  Inverter/1 -> Delay11/1, Delay17/1, Gateway Out7/1
  [slot_ignore] -> Inverter/1
  [new_data] -> ram2/5
  [new_data_we0] -> ram2/6
  [new_data_addr] -> ram2/4
  sync/1 -> Delay16/1, Counter1/1, Register/1, Register/3
  sync_delay/1 -> Delay23/1
  Delay21/1 -> Delay20/1
  Delay20/1 -> sync_out/1
  Mux1/1 -> dout/1
  [readout_buf1] -> Delay25/1
  Delay12/1 -> Mux/1
  [ram0_en] -> Delay22/1
  [new_data_we1] -> ram1/6
  [new_data_addr] -> ram1/4
  [new_data] -> ram1/5
  [ram1_en] -> Delay8/1
  [ram0_en] -> Delay6/1
  ram1/1 -> Mux/2, Mux1/2
  Constant4/1 -> ram2/2
  Constant3/1 -> ram1/2
  Mux3/1 -> ram1/1
  [buf_rd_addr] -> Mux3/3
  [slot_idx] -> Mux3/2
  [slot_idx] -> Mux2/2
  [buf_rd_addr] -> Mux2/3
  Mux2/1 -> ram2/1
  Mux/1 -> [cur_data]
  [readout_buf0] -> Delay24/1
  ram2/1 -> Mux1/3, Mux/3
  Slice2/1 -> Delay5/1
  Delay4/1 -> [new_data_addr]
  bus_addsub/1(dout) -> [new_data]
  Delay3/1 -> Delay4/1
  Delay2/1 -> bus_addsub/1(a)
  [cur_data] -> bus_addsub/2(b)
  Delay1/1 -> Delay2/1
  Slice/1 -> [slot_idx]
  din/1 -> Delay1/1
  Constant2/1 -> map1/3(we)
  Constant1/1 -> map1/2(data_in)
  [vec_idx] -> Gateway Out/1, map1/1(addr)
  Slice1/1 -> Delay18/1, Relational1/1, [vec_idx]
  Counter1/1 -> Slice1/1, Slice2/1
  map1/1(data_out) -> Gateway Out8/1, Slice/1, Slice3/1
  Inverter3/1 -> [ram0_en]
  Constant5/1 -> Relational1/2
  Relational1/1 -> [ignore]
  Inverter1/1 -> [readout_buf1]
  Delay16/1 -> sync_delay/1
  Gateway Out1/1 -> Scope4/1
  ? -> Scope4/3
  Gateway Out3/1 -> Scope4/2
  Gateway Out9/1 -> Scope4/4
  From15/1 -> Gateway Out1/1
  From8/1 -> Gateway Out3/1
  From20/1 -> Gateway Out9/1
  Delay18/1 -> [buf_rd_addr]
  ? -> Scope/3
  Gateway Out/1 -> Scope/1
  ? -> Scope/4
  Gateway Out8/1 -> Scope/2
  Delay19/1 -> Delay10/1
  Delay22/1 -> Delay12/1
  Delay23/1 -> Delay21/1
  Delay24/1 -> ram2/3
  Delay25/1 -> ram1/3

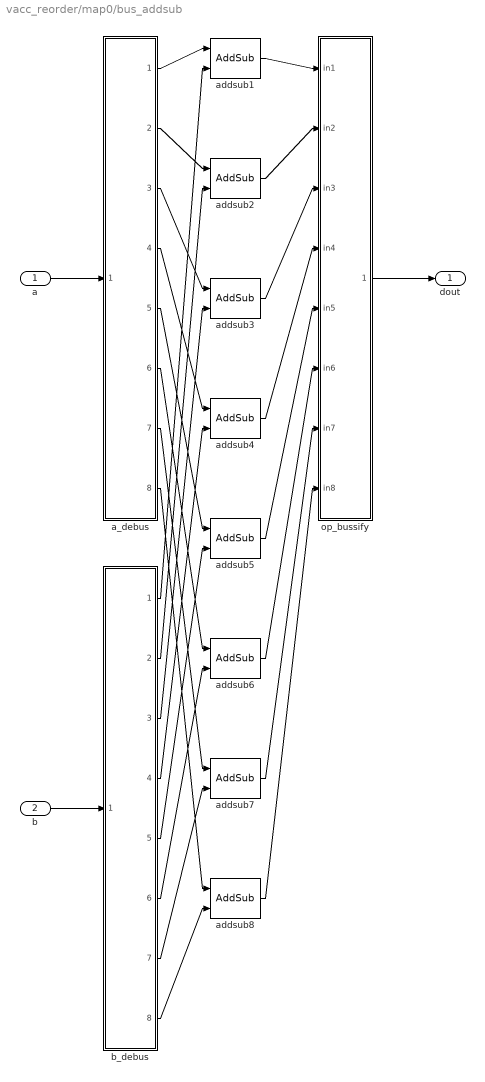
== system vacc_reorder/map0/bus_addsub ==
  a : Inport
  b : Inport  Port=2
  a_debus : Subsystem  AncestorBlock=casper_library_flow_control/bus_expand  mask(bus_expand){mode=divisions of arbitrary size, outputNum=2, outputWidth=[18  18  18  18  18  18  18  18], outputBinaryPt=[0  0  0  0  0  0  0  0], outputArithmeticType=[1  1  1  1  1  1  1  1], show_format=on, outputToWorkspace=off, variablePrefix=, outputToModelAsWell=on}
      mask prompts: outputNum "Number of outputs:"; outputWidth "Output width:"; outputBinaryPt "Output binary point position:"; outputArithmeticType "Output arithmetic type (ufix=0, fix=1, bool=2):"; show_format "Print format string?"; outputToWorkspace "Output to workspace?"; variablePrefix "Variable name prefix:"; outputToModelAsWell "Output to model as well?"
      mask help:
      | Expands a 'bus' made using a bus_create or Xilinx
      | concat block.
      | The input will be divided into the specified number
      | of outputs with the specified arithmetic types.
      | Divisions are made from most significant bit.
      mask init:
      | bus_expand_init(gcb,...
      |     'mode', mode, ...
      |     'outputNum', outputNum, ...
      |     'outputWidth', outputWidth, ...
      |     'outputBinaryPt', outputBinaryPt, ...
      |     'outputArithmeticType', outputArithmeticType, ...
      |     'show_format', show_format, ...
      |     'outputToWorkspace', outputToWorkspace, ...
      |     'variablePrefix', variablePrefix, ...
      |     'outputToModelAsWell', outputToModelAsWell);
      settings: AttributesFormatString=8 outputs: f18.0,f18.0,f18.0,f18.0,f18.0,f18.0,f18.0,f18.0,
      mask TypeOptions mode: divisions of equal size | divisions of arbitrary size
      mask Callback mode: %bus_expand_callback();
      mask Callback outputWidth: %bus_expand_callback();
      mask Callback outputToWorkspace: %bus_expand_callback();
  addsub{1..8} (8 alike) : xbsIndex_r4/AddSub  mode=Addition  use_carryin=off  use_carryout=off  en=off  latency=2  precision=User Defined  arith_type="Signed  (2's comp)"  n_bits=18  bin_pt=0  quantization=Truncate  overflow=Saturate  use_behavioral_HDL=on  hw_selection=Fabric  pipelined=on  dbl_ovrd=off  block_type=addsub
  b_debus : Subsystem  AncestorBlock=casper_library_flow_control/bus_expand  mask(bus_expand){mode=divisions of arbitrary size, outputNum=2, outputWidth=[18  18  18  18  18  18  18  18], outputBinaryPt=[0  0  0  0  0  0  0  0], outputArithmeticType=[1  1  1  1  1  1  1  1], show_format=on, outputToWorkspace=off, variablePrefix=, outputToModelAsWell=on}
      mask prompts: outputNum "Number of outputs:"; outputWidth "Output width:"; outputBinaryPt "Output binary point position:"; outputArithmeticType "Output arithmetic type (ufix=0, fix=1, bool=2):"; show_format "Print format string?"; outputToWorkspace "Output to workspace?"; variablePrefix "Variable name prefix:"; outputToModelAsWell "Output to model as well?"
      mask help:
      | Expands a 'bus' made using a bus_create or Xilinx
      | concat block.
      | The input will be divided into the specified number
      | of outputs with the specified arithmetic types.
      | Divisions are made from most significant bit.
      mask init: same as vacc_reorder/map0/bus_addsub/a_debus
      settings: AttributesFormatString=8 outputs: f18.0,f18.0,f18.0,f18.0,f18.0,f18.0,f18.0,f18.0,
      mask TypeOptions mode: divisions of equal size | divisions of arbitrary size
      mask Callback mode: %bus_expand_callback();
      mask Callback outputWidth: %bus_expand_callback();
      mask Callback outputToWorkspace: %bus_expand_callback();
  op_bussify : Subsystem  AncestorBlock=casper_library_flow_control/bus_create  mask(bus_create){inputNum=8}
      mask prompts: inputNum "Number of inputs:"
      mask init:
      | bus_create_init(gcb,...
      |     'inputNum', inputNum);
  dout : Outport
  wires:
  op_bussify/1(bus_out) -> dout/1
  addsub8/1 -> op_bussify/8(in8)
  addsub7/1 -> op_bussify/7(in7)
  addsub6/1 -> op_bussify/6(in6)
  addsub5/1 -> op_bussify/5(in5)
  addsub4/1 -> op_bussify/4(in4)
  addsub3/1 -> op_bussify/3(in3)
  addsub2/1 -> op_bussify/2(in2)
  addsub1/1 -> op_bussify/1(in1)
  b_debus/8(lsb_out1) -> addsub8/2
  a_debus/8(lsb_out1) -> addsub8/1
  b_debus/7(out2) -> addsub7/2
  a_debus/7(out2) -> addsub7/1
  b_debus/6(out3) -> addsub6/2
  a_debus/6(out3) -> addsub6/1
  b_debus/5(out4) -> addsub5/2
  a_debus/5(out4) -> addsub5/1
  b_debus/4(out5) -> addsub4/2
  a_debus/4(out5) -> addsub4/1
  b_debus/3(out6) -> addsub3/2
  a_debus/3(out6) -> addsub3/1
  b_debus/2(out7) -> addsub2/2
  a_debus/2(out7) -> addsub2/1
  b_debus/1(msb_out8) -> addsub1/2
  a_debus/1(msb_out8) -> addsub1/1
  b/1 -> b_debus/1(bus_in)
  a/1 -> a_debus/1(bus_in)
